simulink model "A3_Multi_DC_bus"  (R2022b)
settings: Solver=ode4  StartTime=0.0  StopTime=tdist2  FixedStep=ts  RelTol=1e-3
undefined symbols (not defined in the file): C, C_bc_ESS, C_bc_PV, C_bc_SC, C_SC_set, Cf, f0, fc, fc1, fv, Gf, Idcbase, Idcbase1, Idcbase2, Ilim, J, Ki_c1, Ki_v, Kp_c1, Kp_v, L_bc_ESS, L_bc_PV, L_bc_SC, L_line_ESS, L_line_PV, Lf, Plim_ESS, Plim_PV, Plim_PV1, Plim_PV2, Plim_SC, Pnom, Pset_ESS, Pset_inv, Pset_load, Pset_PV, Pset_PV1, Pset_PV2, Pset_SC, Qset_inv, R1_line_PV, R2_line_PV, R_bc_ESS, R_bc_PV, R_bc_SC, R_line_ESS, R_line_PV, R_line_SC, Rf, Rg, Sbase, sps, Stotal, tdist1, tdist2, tESSconnect, tPVconnect, ts, tSCconnect, V1 ... (+19)
libraries: spsSeriesRLCBranchLib x20, spsVoltageMeasurementLib x12, spsCurrentMeasurementLib x10, cstblocks x10, spsControlledVoltageSourceLib x9, spsPWMGeneratorDCDCLib x5, spsTwoQuadrantDCDCConverterLib x5, simulink_extras x5, spsBreakerLib x4, spsThreePhaseVIMeasurementLib x3, spsabctoAlphaBetaZeroLib x3, spsThreePhaseSeriesRLCBranchLib x3
(part 2 of 2)

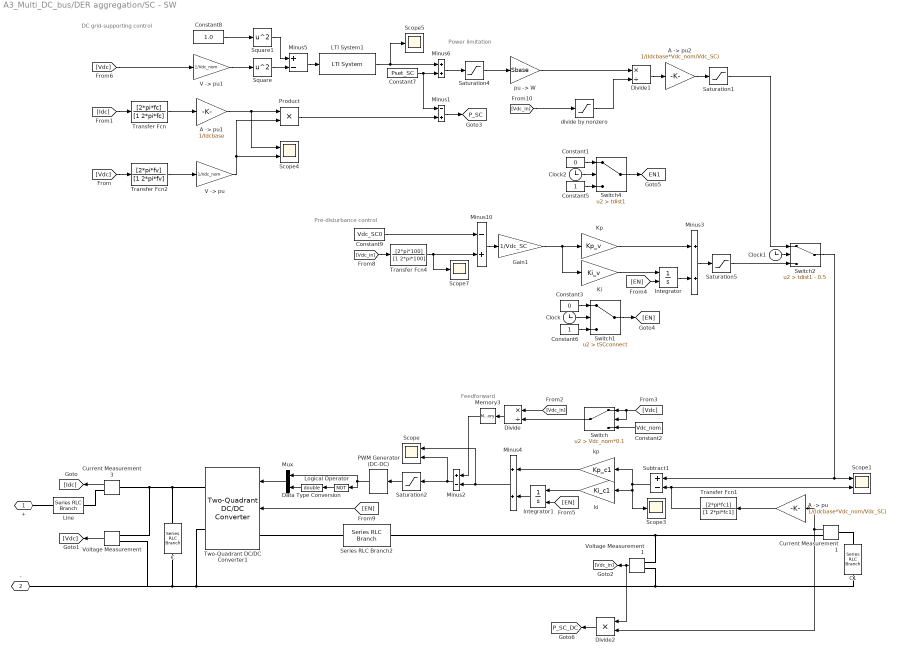
== system A3_Multi_DC_bus/DER aggregation/SC - SW ==
  note: Power limitation
  note: Pre-disturbance control
  note: DC grid-supporting control
  note: Feedforward
  "A -> pu" : Gain  Gain=1/(Idcbase*Vdc_nom/Vdc_SC)
  "A -> pu1" : Gain  Gain=1/Idcbase
  "A -> pu2" : Gain  Gain=1/(Idcbase*Vdc_nom/Vdc_SC)
  C : spsSeriesRLCBranchLib/Series RLC Branch  LConnTagsString=__new0  RConnTagsString=__new0  BranchType=C  Resistance=0.001  Inductance=L_line_PV  SetiL0=off  InitialCurrent=0  Capacitance=C_bc_SC  Setx0=on  InitialVoltage=Vdc_nom  Measurements=None
  C1 : spsSeriesRLCBranchLib/Series RLC Branch  LConnTagsString=__new0  RConnTagsString=__new0  BranchType=C  Resistance=0.001  Inductance=L_line_PV  SetiL0=off  InitialCurrent=0  Capacitance=C_SC_set  Setx0=on  InitialVoltage=Vdc_SC0  Measurements=None
  Clock : Clock
  Clock1 : Clock
  Clock2 : Clock
  Constant1 : Constant  Value=0
  Constant2 : Constant  Value=Vdc_nom
  Constant3 : Constant  Value=0
  Constant5 : Constant
  Constant6 : Constant
  Constant7 : Constant  Value=Pset_SC
  Constant8 : Constant  Value=1.0
  Constant9 : Constant  Value=Vdc_SC0
  Current Measurement1 : spsCurrentMeasurementLib/Current Measurement  PhasorSimulation=off  OutputType=Complex  PSBequivalent=0
  Current Measurement3 : spsCurrentMeasurementLib/Current Measurement  PhasorSimulation=off  OutputType=Complex  PSBequivalent=0
  Data Type Conversion : DataTypeConversion  OutDataTypeStr=double  SaturateOnIntegerOverflow=off  RndMeth=Floor
  Divide : Product  Inputs=*/
  Divide1 : Product  Inputs=*/
  Divide2 : Product  Inputs=**
  Gain1 : Gain  Gain=1/Vdc_SC
  Integrator : Integrator  ExternalReset=level hold  UpperSaturationLimit=1.5  LowerSaturationLimit=-0.5
  Integrator1 : Integrator  ExternalReset=level hold  LimitOutput=on  UpperSaturationLimit=1  LowerSaturationLimit=-1
  Ki : Gain  Gain=Ki_v
  Kp : Gain  Gain=Kp_v
  LTI System1 : cstblocks/LTI System  sys=T_SC1  IC=[]
  Line : spsSeriesRLCBranchLib/Series RLC Branch  LConnTagsString=__new0  RConnTagsString=__new0  BranchType=R  Resistance=R_line_SC  Inductance=L_line_ESS  SetiL0=off  InitialCurrent=0  Capacitance=1e-6  Setx0=off  InitialVoltage=0  Measurements=None
  Logical Operator : Logic  Operator=NOT  AllPortsSameDT=off  OutDataTypeStr=boolean
  Memory3 : Memory
  Minus1 : Sum  Inputs=-+
  Minus10 : Sum  Inputs=-+
  Minus2 : Sum  Inputs=+-
  Minus3 : Sum
  Minus4 : Sum
  Minus5 : Sum  Inputs=+-
  Minus6 : Sum
  Mux : Mux  Inputs=2
  PWM Generator (DC-DC) : spsPWMGeneratorDCDCLib/PWM Generator (DC-DC)  Fsw=fw  Ts=0
  Product : Product
  Saturation1 : Saturate  UpperLimit=1.0  LowerLimit=-1.0
  Saturation2 : Saturate  UpperLimit=1  LowerLimit=0
  Saturation4 : Saturate  UpperLimit=Plim_SC  LowerLimit=-Plim_SC
  Saturation5 : Saturate  UpperLimit=1.0  LowerLimit=-1.0
  Scope : Scope  NumInputPorts=2
  Scope1 : Scope  NumInputPorts=2
  Scope3 : Scope
  Scope4 : Scope  NumInputPorts=2
  Scope5 : Scope
  Scope7 : Scope
  Series RLC Branch2 : spsSeriesRLCBranchLib/Series RLC Branch  LConnTagsString=__new0  RConnTagsString=__new0  BranchType=RL  Resistance=R_bc_SC  Inductance=L_bc_SC  SetiL0=off  InitialCurrent=Pset_SC*Idcbase*Vdc_nom/Vdc_PV  Capacitance=1e-6  Setx0=off  InitialVoltage=0  Measurements=None
  Square : Math  Operator=square
  Square1 : Math  Operator=square
  Subtract1 : Sum  Inputs=+-
  Switch : Switch  Criteria=u2 > Threshold  Threshold=Vdc_nom*0.1  SaturateOnIntegerOverflow=off  InputSameDT=off
  Switch1 : Switch  Criteria=u2 > Threshold  Threshold=tSCconnect  SaturateOnIntegerOverflow=off  InputSameDT=off
  Switch2 : Switch  Criteria=u2 > Threshold  Threshold=tdist1 - 0.5  SaturateOnIntegerOverflow=off  InputSameDT=off
  Switch4 : Switch  Criteria=u2 > Threshold  Threshold=tdist1  SaturateOnIntegerOverflow=off  InputSameDT=off
  Transfer Fcn : TransferFcn  Numerator=[2*pi*fc]  Denominator=[1 2*pi*fc]
  Transfer Fcn1 : TransferFcn  Numerator=[2*pi*fc1]  Denominator=[1 2*pi*fc1]
  Transfer Fcn2 : TransferFcn  Numerator=[2*pi*fv]  Denominator=[1 2*pi*fv]
  Transfer Fcn4 : TransferFcn  Numerator=[2*pi*100]  Denominator=[1 2*pi*100]
  Two-Quadrant DC/DC Converter1 : spsTwoQuadrantDCDCConverterLib/Two-Quadrant DC//DC Converter  ModelType=Switching devices  Ron=1e-4  Rs=1e6  Cs=inf  Vforward=[0,0]  Ron_Diode=1e-3  Rs_Diode=1e6  Cs_Diode=inf  Vf_Diode=1e-3  Rs_CurrentSource=inf  Ron_ACsource=1e-3
      settings: LibrarySourceBlock=|
      | sps_lib/Power Electronics/Two-Quadrant
      | DC//DC Converter
  "V -> pu" : Gain  Gain=1/Vdc_nom
  "V -> pu1" : Gain  Gain=1/Vdc_nom
  Voltage Measurement : spsVoltageMeasurementLib/Voltage Measurement  PhasorSimulation=off  OutputType=Complex  PSBequivalent=0
  Voltage Measurement1 : spsVoltageMeasurementLib/Voltage Measurement  PhasorSimulation=off  OutputType=Complex  PSBequivalent=0
  divide by nonzero : Saturate  UpperLimit=1e6  LowerLimit=1e-6
  ki : Gain  Gain=Ki_c1
  kp : Gain  Gain=Kp_c1
  "pu -> W" : Gain  Gain=Sbase
  + : PMIOPort  Side=Left
  - : PMIOPort  Port=2  Side=Right
  tag scope: EN1=global, P_SC=global, P_SC_DC=global
  wires:
  Constant1/1 -> Switch4/1
  Switch4/1 -> [EN1]
  Clock2/1 -> Switch4/2
  Constant5/1 -> Switch4/3
  Saturation5/1 -> Switch2/3
  Minus1/1 -> [P_SC]
  Saturation4/1 -> "pu -> W"/1
  Subtract1/1 -> ki/1, Scope3/1, kp/1
  Minus6/1 -> Saturation4/1
  Divide1/1 -> "A -> pu2"/1
  divide by nonzero/1 -> Divide1/2
  "pu -> W"/1 -> Divide1/1
  "A -> pu2"/1 -> Saturation1/1
  Clock1/1 -> Switch2/2
  Minus10/1 -> Gain1/1
  [Vdc_in] -> Transfer Fcn4/1
  Constant9/1 -> Minus10/1
  Transfer Fcn4/1 -> Minus10/2, Scope7/1
  [Idc] -> Transfer Fcn/1
  Voltage Measurement/1 -> [Vdc]
  Current Measurement3/1 -> [Idc]
  [EN] -> Two-Quadrant DC/DC Converter1/2
  Current Measurement1/1 -> Divide2/2, "A -> pu"/1
  Transfer Fcn1/1 -> Subtract1/2, Scope1/2
  Product/1 -> Minus1/2
  Switch/1 -> Divide/2
  Constant2/1 -> Switch/3
  [Vdc_in] -> Divide/1
  Divide/1 -> Memory3/1
  Voltage Measurement1/1 -> Divide2/1, [Vdc_in]
  [Vdc] -> Switch/2, Switch/1
  Minus3/1 -> Saturation5/1
  Saturation1/1 -> Switch2/1
  Ki/1 -> Integrator/1
  Integrator/1 -> Minus3/2
  Kp/1 -> Minus3/1
  kp/1 -> Minus4/1
  Integrator1/1 -> Minus4/2
  ki/1 -> Integrator1/1
  Clock/1 -> Switch1/2
  Switch1/1 -> [EN]
  Constant3/1 -> Switch1/1
  Constant6/1 -> Switch1/3
  [EN] -> Integrator/2
  [EN] -> Integrator1/2
  Constant8/1 -> Square1/1
  Square/1 -> Minus5/2
  Square1/1 -> Minus5/1
  Minus5/1 -> LTI System1/1
  Constant7/1 -> Minus6/2, Minus1/1
  LTI System1/1 -> Minus6/1, Scope5/1
  [Vdc] -> "V -> pu1"/1
  "V -> pu1"/1 -> Square/1
  "V -> pu"/1 -> Product/2, Scope4/2
  "A -> pu1"/1 -> Scope4/1, Product/1
  [Vdc] -> Transfer Fcn2/1
  Minus4/1 -> Minus2/2, Scope/1
  Gain1/1 -> Kp/1, Ki/1
  Minus2/1 -> Scope/2, Saturation2/1
  Transfer Fcn/1 -> "A -> pu1"/1
  Transfer Fcn2/1 -> "V -> pu"/1
  "A -> pu"/1 -> Transfer Fcn1/1
  Memory3/1 -> Minus2/1
  Data Type Conversion/1 -> Mux/2
  Saturation2/1 -> PWM Generator (DC-DC)/1
  PWM Generator (DC-DC)/1 -> Mux/1, Logical Operator/1
  Logical Operator/1 -> Data Type Conversion/1
  Mux/1 -> Two-Quadrant DC/DC Converter1/1
  [Vdc_in] -> divide by nonzero/1
  Divide2/1 -> [P_SC_DC]
  Switch2/1 -> Subtract1/1, Scope1/1
  connections:
  C/RConn1 -- -/RConn1 -- Voltage Measurement/LConn2 -- Two-Quadrant DC/DC Converter1/RConn2 -- C1/RConn1 -- Voltage Measurement1/LConn2
  Two-Quadrant DC/DC Converter1/LConn1 -- Series RLC Branch2/LConn1
  C1/LConn1 -- Current Measurement1/LConn1
  Series RLC Branch2/RConn1 -- Voltage Measurement1/LConn1 -- Current Measurement1/RConn1
  Current Measurement3/RConn1 -- Line/RConn1
  Current Measurement3/LConn1 -- Voltage Measurement/LConn1 -- Two-Quadrant DC/DC Converter1/RConn1 -- C/LConn1
  Line/LConn1 -- +/RConn1

== system A3_Multi_DC_bus/Desired (using causalized Ti)/Int ==
  In : Inport
  Constant6 : Constant  Value=2*pi
  Initial : InitialCondition  Value=0
  Integrator1 : Integrator  ExternalReset=rising  InitialConditionSource=external  InitialCondition=sps.Phase_Init*pi/180  ShowStatePort=on
  Relational Operator : RelationalOperator  Operator=>  OutDataTypeStr=boolean  InputSameDT=off
  Subtract : Sum  Inputs=+-
  wt : Outport
  wires:
  Integrator1/1 -> wt/1
  Initial/1 -> Integrator1/3
  In/1 -> Integrator1/1
  Relational Operator/1 -> Integrator1/2
  Subtract/1 -> Initial/1
  Integrator1/State -> Relational Operator/1, Subtract/1
  Constant6/1 -> Relational Operator/2, Subtract/2

== system A3_Multi_DC_bus/Desired (using causalized Ti)/Inv Tr ==
  wt : Inport
  dq : Inport  Port=2
  Fcn : Fcn  Expr=u[1]*cos(u[3]) - u[2]*sin(u[3])
  Fcn1 : Fcn  Expr=u[1]*sin(u[3]) + u[2]*cos(u[3])
  Mux : Mux  Inputs=2
  Mux2 : Mux  Inputs=[2 1]
  Mux3 : Mux  Inputs=[2 1]
  albe : Outport
  wires:
  Fcn1/1 -> Mux/2
  wt/1 -> Mux2/2, Mux3/2
  Fcn/1 -> Mux/1
  Mux/1 -> albe/1
  dq/1 -> Mux2/1, Mux3/1
  Mux2/1 -> Fcn/1
  Mux3/1 -> Fcn1/1

== system A3_Multi_DC_bus/Subsystem/Int ==
  In : Inport
  Constant6 : Constant  Value=2*pi
  Initial : InitialCondition  Value=0
  Integrator1 : Integrator  ExternalReset=rising  InitialConditionSource=external  InitialCondition=sps.Phase_Init*pi/180  ShowStatePort=on
  Relational Operator : RelationalOperator  Operator=>  OutDataTypeStr=boolean  InputSameDT=off
  Subtract : Sum  Inputs=+-
  Out : Outport
  wires:
  Integrator1/1 -> Out/1
  Initial/1 -> Integrator1/3
  In/1 -> Integrator1/1
  Relational Operator/1 -> Integrator1/2
  Subtract/1 -> Initial/1
  Integrator1/State -> Relational Operator/1, Subtract/1
  Constant6/1 -> Relational Operator/2, Subtract/2

== system A3_Multi_DC_bus/Subsystem2/Int ==
  In : Inport
  Constant6 : Constant  Value=2*pi
  Initial : InitialCondition  Value=0
  Integrator1 : Integrator  ExternalReset=rising  InitialConditionSource=external  InitialCondition=sps.Phase_Init*pi/180  ShowStatePort=on
  Relational Operator : RelationalOperator  Operator=>  OutDataTypeStr=boolean  InputSameDT=off
  Subtract : Sum  Inputs=+-
  Out : Outport
  wires:
  Integrator1/1 -> Out/1
  Initial/1 -> Integrator1/3
  In/1 -> Integrator1/1
  Relational Operator/1 -> Integrator1/2
  Subtract/1 -> Initial/1
  Integrator1/State -> Relational Operator/1, Subtract/1
  Constant6/1 -> Relational Operator/2, Subtract/2

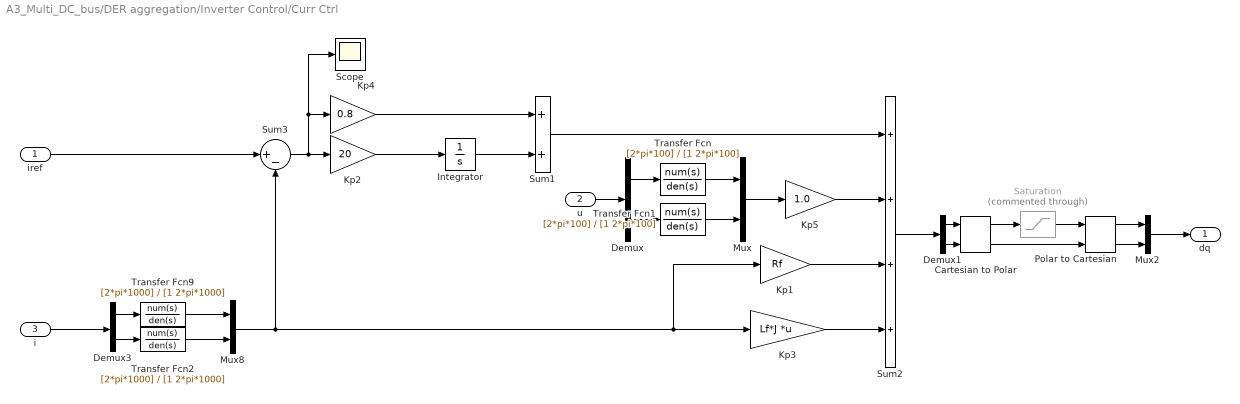
== system A3_Multi_DC_bus/DER aggregation/Inverter Control/Curr Ctrl ==
  iref : Inport
  "u " : Inport  Port=2
  i : Inport  Port=3
  Cartesian to Polar : simulink_extras/Transformations/Cartesian to Polar
  Demux : Demux  Outputs=2
  Demux1 : Demux  Outputs=2
  Demux3 : Demux  Outputs=2
  Integrator : Integrator  InitialCondition=[1 0]
  Kp1 : Gain  Gain=Rf  SaturateOnIntegerOverflow=on  OutDataTypeStr=Inherit: Same as input  ParamDataTypeStr=Inherit: Same as input
  Kp2 : Gain  Gain=20  SaturateOnIntegerOverflow=on  OutDataTypeStr=Inherit: Same as input  ParamDataTypeStr=Inherit: Same as input
  Kp3 : Gain  Gain=Lf*J  Multiplication=Matrix(K*u)  SaturateOnIntegerOverflow=on  OutDataTypeStr=Inherit: Same as input  ParamDataTypeStr=Inherit: Same as input
  Kp4 : Gain  Gain=0.8  SaturateOnIntegerOverflow=on  OutDataTypeStr=Inherit: Same as input  ParamDataTypeStr=Inherit: Same as input
  Kp5 : Gain  Gain=1.0  SaturateOnIntegerOverflow=on  OutDataTypeStr=Inherit: Same as input  ParamDataTypeStr=Inherit: Same as input
  Mux : Mux  Inputs=2
  Mux2 : Mux  Inputs=2
  Mux8 : Mux  Inputs=2
  Polar to Cartesian : simulink_extras/Transformations/Polar to Cartesian
  Saturation : Saturate  Commented=through  UpperLimit=1.5  LowerLimit=0
  Scope : Scope
  Sum1 : Sum
  Sum2 : Sum  Inputs=++++
  Sum3 : Sum  Inputs=|+-
  Transfer Fcn : TransferFcn  Numerator=[2*pi*100]  Denominator=[1 2*pi*100]
  Transfer Fcn1 : TransferFcn  Numerator=[2*pi*100]  Denominator=[1 2*pi*100]
  Transfer Fcn2 : TransferFcn  Numerator=[2*pi*1000]  Denominator=[1 2*pi*1000]
  Transfer Fcn9 : TransferFcn  Numerator=[2*pi*1000]  Denominator=[1 2*pi*1000]
  dq : Outport
  wires:
  Demux3/2 -> Transfer Fcn2/1
  i/1 -> Demux3/1
  Demux3/1 -> Transfer Fcn9/1
  Transfer Fcn9/1 -> Mux8/1
  Transfer Fcn2/1 -> Mux8/2
  iref/1 -> Sum3/1
  Saturation/1 -> Polar to Cartesian/1
  Polar to Cartesian/1 -> Mux2/1
  Sum2/1 -> Demux1/1
  Demux1/1 -> Cartesian to Polar/1
  Cartesian to Polar/1 -> Saturation/1
  Cartesian to Polar/2 -> Polar to Cartesian/2
  Polar to Cartesian/2 -> Mux2/2
  Demux1/2 -> Cartesian to Polar/2
  Transfer Fcn/1 -> Mux/1
  Transfer Fcn1/1 -> Mux/2
  Demux/2 -> Transfer Fcn1/1
  Demux/1 -> Transfer Fcn/1
  Mux/1 -> Kp5/1
  Kp5/1 -> Sum2/2
  "u "/1 -> Demux/1
  Kp3/1 -> Sum2/4
  Kp1/1 -> Sum2/3
  Mux2/1 -> dq/1
  Kp2/1 -> Integrator/1
  Mux8/1 -> Kp3/1, Kp1/1, Sum3/2
  Integrator/1 -> Sum1/2
  Kp4/1 -> Sum1/1
  Sum3/1 -> Kp2/1, Kp4/1, Scope/1
  Sum1/1 -> Sum2/1

== system A3_Multi_DC_bus/DER aggregation/Inverter Control/Curr T ==
  abc : Inport
  In2 : Inport  Port=2
  Demux : Demux  Outputs=3
  Mux1 : Mux  Inputs=2
  Subsystem : Subsystem
  Terminator2 : Terminator
  abc to Alpha-Beta-Zero : spsabctoAlphaBetaZeroLib/abc to Alpha-Beta-Zero
  dq : Outport
  wires:
  In2/1 -> Subsystem/2(wt)
  Mux1/1 -> Subsystem/1(albe)
  abc/1 -> abc to Alpha-Beta-Zero/1
  Demux/2 -> Mux1/2
  Demux/1 -> Mux1/1
  Demux/3 -> Terminator2/1
  abc to Alpha-Beta-Zero/1 -> Demux/1
  Subsystem/1(dq) -> dq/1

== system A3_Multi_DC_bus/DER aggregation/Inverter Control/Curr in T ==
  abc : Inport
  In2 : Inport  Port=2
  Demux : Demux  Outputs=3
  Mux1 : Mux  Inputs=2
  Subsystem : Subsystem
  Terminator2 : Terminator
  abc to Alpha-Beta-Zero : spsabctoAlphaBetaZeroLib/abc to Alpha-Beta-Zero
  dq : Outport
  wires:
  Subsystem/1(dq) -> dq/1
  In2/1 -> Subsystem/2(wt)
  Mux1/1 -> Subsystem/1(albe)
  abc/1 -> abc to Alpha-Beta-Zero/1
  Demux/2 -> Mux1/2
  Demux/1 -> Mux1/1
  Demux/3 -> Terminator2/1
  abc to Alpha-Beta-Zero/1 -> Demux/1

== system A3_Multi_DC_bus/DER aggregation/Inverter Control/Int ==
  In : Inport
  Constant6 : Constant  Value=2*pi
  Initial : InitialCondition  Value=0
  Integrator1 : Integrator  ExternalReset=rising  InitialConditionSource=external  InitialCondition=sps.Phase_Init*pi/180  ShowStatePort=on
  Relational Operator : RelationalOperator  Operator=>  OutDataTypeStr=boolean  InputSameDT=off
  Subtract : Sum  Inputs=+-
  Out : Outport
  wires:
  Integrator1/1 -> Out/1
  Initial/1 -> Integrator1/3
  In/1 -> Integrator1/1
  Relational Operator/1 -> Integrator1/2
  Subtract/1 -> Initial/1
  Integrator1/State -> Relational Operator/1, Subtract/1
  Constant6/1 -> Relational Operator/2, Subtract/2

== system A3_Multi_DC_bus/DER aggregation/Inverter Control/Inv Tr ==
  dq : Inport
  wt : Inport  Port=2
  Fcn : Fcn  Expr=u[1]*cos(u[3]) - u[2]*sin(u[3])
  Fcn1 : Fcn  Expr=u[1]*sin(u[3]) + u[2]*cos(u[3])
  Mux : Mux  Inputs=2
  Mux2 : Mux  Inputs=[2 1]
  Mux3 : Mux  Inputs=[2 1]
  albe : Outport
  wires:
  Fcn1/1 -> Mux/2
  wt/1 -> Mux2/2, Mux3/2
  Fcn/1 -> Mux/1
  Mux/1 -> albe/1
  dq/1 -> Mux2/1, Mux3/1
  Mux2/1 -> Fcn/1
  Mux3/1 -> Fcn1/1

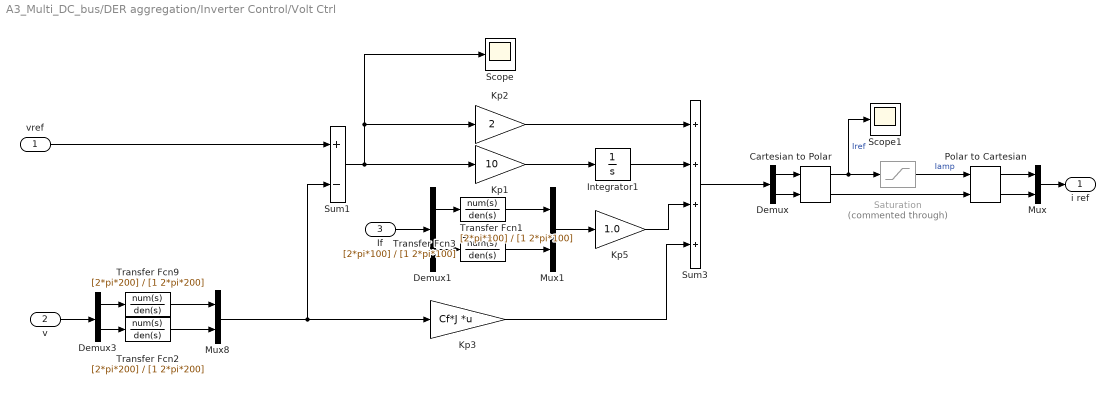
== system A3_Multi_DC_bus/DER aggregation/Inverter Control/Volt Ctrl ==
  vref : Inport
  v : Inport  Port=2
  If : Inport  Port=3
  Cartesian to Polar : simulink_extras/Transformations/Cartesian to Polar
  Demux : Demux  Outputs=2
  Demux1 : Demux  Outputs=2
  Demux3 : Demux  Outputs=2
  Integrator1 : Integrator  InitialCondition=[0 0]
  Kp1 : Gain  Gain=10  SaturateOnIntegerOverflow=on  OutDataTypeStr=Inherit: Same as input  ParamDataTypeStr=Inherit: Same as input
  Kp2 : Gain  Gain=2  SaturateOnIntegerOverflow=on  OutDataTypeStr=Inherit: Same as input  ParamDataTypeStr=Inherit: Same as input
  Kp3 : Gain  Gain=Cf*J  Multiplication=Matrix(K*u)  SaturateOnIntegerOverflow=on  OutDataTypeStr=Inherit: Same as input  ParamDataTypeStr=Inherit: Same as input
  Kp5 : Gain  Gain=1.0  SaturateOnIntegerOverflow=on  OutDataTypeStr=Inherit: Same as input  ParamDataTypeStr=Inherit: Same as input
  Mux : Mux  Inputs=2
  Mux1 : Mux  Inputs=2
  Mux8 : Mux  Inputs=2
  Polar to Cartesian : simulink_extras/Transformations/Polar to Cartesian
  Saturation : Saturate  Commented=through  UpperLimit=Ilim  LowerLimit=0
  Scope : Scope
  Scope1 : Scope
  Sum1 : Sum  Inputs=+-
  Sum3 : Sum  Inputs=++++
  Transfer Fcn1 : TransferFcn  Numerator=[2*pi*100]  Denominator=[1 2*pi*100]
  Transfer Fcn2 : TransferFcn  Numerator=[2*pi*200]  Denominator=[1 2*pi*200]
  Transfer Fcn3 : TransferFcn  Numerator=[2*pi*100]  Denominator=[1 2*pi*100]
  Transfer Fcn9 : TransferFcn  Numerator=[2*pi*200]  Denominator=[1 2*pi*200]
  i ref : Outport
  wires:
  vref/1 -> Sum1/1
  Demux1/2 -> Transfer Fcn3/1
  Demux/1 -> Cartesian to Polar/1
  Mux8/1 -> Sum1/2, Kp3/1
  Cartesian to Polar/2 -> Polar to Cartesian/2
  Demux/2 -> Cartesian to Polar/2
  Saturation/1 -> Polar to Cartesian/1  "Iamp"
  Integrator1/1 -> Sum3/2
  Mux1/1 -> Kp5/1
  Kp1/1 -> Integrator1/1
  Transfer Fcn1/1 -> Mux1/1
  Kp2/1 -> Sum3/1
  Transfer Fcn3/1 -> Mux1/2
  If/1 -> Demux1/1
  Demux1/1 -> Transfer Fcn1/1
  Kp5/1 -> Sum3/3
  Sum3/1 -> Demux/1
  Sum1/1 -> Kp2/1, Scope/1, Kp1/1
  Polar to Cartesian/1 -> Mux/1
  Polar to Cartesian/2 -> Mux/2
  Mux/1 -> i ref/1
  Cartesian to Polar/1 -> Saturation/1, Scope1/1  "Iref"
  Transfer Fcn2/1 -> Mux8/2
  Transfer Fcn9/1 -> Mux8/1
  Demux3/2 -> Transfer Fcn2/1
  Demux3/1 -> Transfer Fcn9/1
  v/1 -> Demux3/1
  Kp3/1 -> Sum3/4

== system A3_Multi_DC_bus/DER aggregation/Inverter Control/Volt T ==
  abc : Inport
  In2 : Inport  Port=2
  Demux : Demux  Outputs=3
  Mux1 : Mux  Inputs=2
  Subsystem : Subsystem
  Terminator2 : Terminator
  abc to Alpha-Beta-Zero : spsabctoAlphaBetaZeroLib/abc to Alpha-Beta-Zero
  dq : Outport
  wires:
  Subsystem/1(dq) -> dq/1
  abc to Alpha-Beta-Zero/1 -> Demux/1
  Demux/3 -> Terminator2/1
  Demux/1 -> Mux1/1
  Demux/2 -> Mux1/2
  abc/1 -> abc to Alpha-Beta-Zero/1
  Mux1/1 -> Subsystem/1(albe)
  In2/1 -> Subsystem/2(wt)

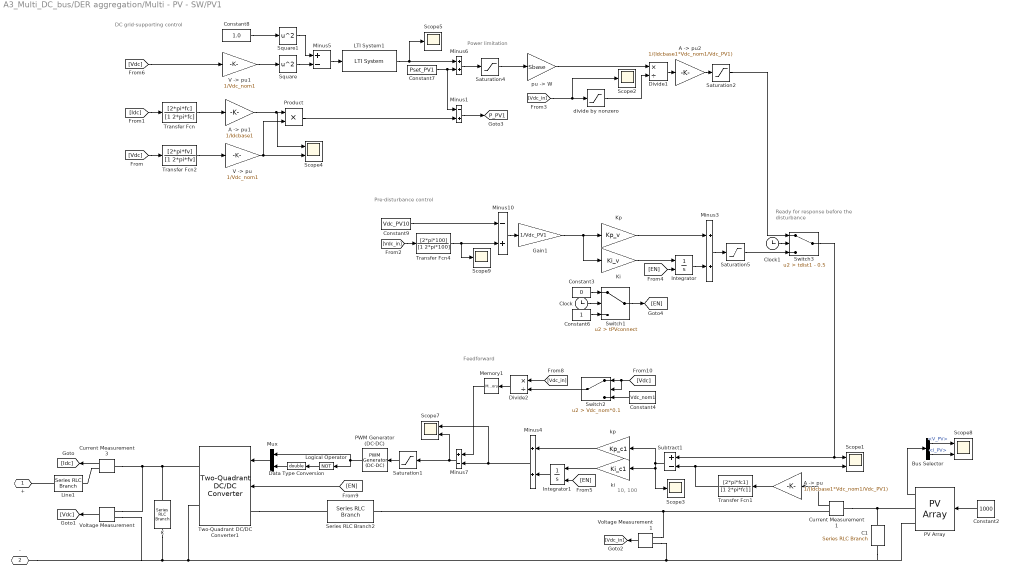
== system A3_Multi_DC_bus/DER aggregation/Multi - PV - SW/PV1 ==
  note: Ready for response
      | before the disturbance
  note: Feedforward
  note: DC grid-supporting control
  note: 10, 100
  note: Pre-disturbance control
  note: Power limitation
  "A -> pu" : Gain  Gain=1/(Idcbase1*Vdc_nom1/Vdc_PV1)
  "A -> pu1" : Gain  Gain=1/Idcbase1
  "A -> pu2" : Gain  Gain=1/(Idcbase1*Vdc_nom1/Vdc_PV1)
  Bus Selector : BusSelector  OutputSignals=V_PV,I_PV
  C : spsSeriesRLCBranchLib/Series RLC Branch  LConnTagsString=__new0  RConnTagsString=__new0  BranchType=C  Resistance=0.001  Inductance=L_line_PV  SetiL0=off  InitialCurrent=0  Capacitance=C_bc_PV  Setx0=on  InitialVoltage=Vdc_nom1  Measurements=None
  C1 : spsSeriesRLCBranchLib/Series RLC Branch  LConnTagsString=__new0  RConnTagsString=__new0  BranchType=C  Resistance=0.001  Inductance=L_line_PV  SetiL0=off  InitialCurrent=0  Capacitance=C_bc_PV  Setx0=on  InitialVoltage=Vdc_PV10  Measurements=None
  Clock : Clock
  Clock1 : Clock
  Constant2 : Constant  Value=1000
  Constant3 : Constant  Value=0
  Constant4 : Constant  Value=Vdc_nom1
  Constant6 : Constant
  Constant7 : Constant  Value=Pset_PV1
  Constant8 : Constant  Value=1.0
  Constant9 : Constant  Value=Vdc_PV10
  Current Measurement1 : spsCurrentMeasurementLib/Current Measurement  PhasorSimulation=off  OutputType=Complex  PSBequivalent=0
  Current Measurement3 : spsCurrentMeasurementLib/Current Measurement  PhasorSimulation=off  OutputType=Complex  PSBequivalent=0
  Data Type Conversion : DataTypeConversion  OutDataTypeStr=double  SaturateOnIntegerOverflow=off  RndMeth=Floor
  Divide1 : Product  Inputs=*/
  Divide2 : Product  Inputs=*/
  Gain1 : Gain  Gain=1/Vdc_PV1
  Integrator : Integrator  ExternalReset=level hold  UpperSaturationLimit=1.5  LowerSaturationLimit=-0.5
  Integrator1 : Integrator  ExternalReset=level hold  LimitOutput=on  UpperSaturationLimit=1  LowerSaturationLimit=-1
  Ki : Gain  Gain=Ki_v
  Kp : Gain  Gain=Kp_v
  LTI System1 : cstblocks/LTI System  sys=T_PV1  IC=[]
  Line1 : spsSeriesRLCBranchLib/Series RLC Branch  LConnTagsString=__new0  RConnTagsString=__new0  BranchType=R  Resistance=R1_line_PV  Inductance=L_line_PV  SetiL0=off  InitialCurrent=0  Capacitance=1e-6  Setx0=off  InitialVoltage=0  Measurements=None
  Logical Operator : Logic  Operator=NOT  AllPortsSameDT=off  OutDataTypeStr=boolean
  Memory1 : Memory
  Minus1 : Sum  Inputs=-+
  Minus10 : Sum  Inputs=-+
  Minus3 : Sum
  Minus4 : Sum
  Minus5 : Sum  Inputs=+-
  Minus6 : Sum
  Minus7 : Sum  Inputs=+-
  Mux : Mux  Inputs=2
  PV Array : spsPVArrayLib/PV Array  Npar=408  Nser=4  PlotType=array @ 1000 W/m2 & specified temperatures  S_vec="[ 1000  500  100 ]"  Temp_C_vec=40  ModuleName=SunPower SPR-315E-WHT-D  PlotWhenSelected=off  Pm=315.072  Ncell=96  Voc=64.6  Isc=6.14  Vm=54.7  Im=5.76  beta_Voc_pc=-0.2727  alpha_Isc_pc=0.061743  beta_Voc=-0.17616  alpha_Isc=0.003791  IL=6.1461  I0=6.5067e-12  nI=0.95071  Rsh=430.0666  Rs=0.43041  RobustModel=on  RobustCellTemperature=40  BAL=off  Tc=1e-6  Tfilter=5e-5
  PWM Generator (DC-DC) : spsPWMGeneratorDCDCLib/PWM Generator (DC-DC)  Fsw=fw  Ts=0
  Product : Product
  Saturation1 : Saturate  UpperLimit=1  LowerLimit=0
  Saturation2 : Saturate  UpperLimit=1.0  LowerLimit=-1.0
  Saturation4 : Saturate  UpperLimit=Plim_PV1  LowerLimit=0
  Saturation5 : Saturate  UpperLimit=1.0  LowerLimit=-1.0
  Scope{1,4,7..8} (4 alike) : Scope  NumInputPorts=2
  Scope{2..3,5,9} (4 alike) : Scope
  Series RLC Branch2 : spsSeriesRLCBranchLib/Series RLC Branch  LConnTagsString=__new0  RConnTagsString=__new0  BranchType=RL  Resistance=R_bc_PV  Inductance=L_bc_PV  SetiL0=off  InitialCurrent=Pset_PV*Idcbase*Vdc_nom/Vdc_PV  Capacitance=1e-6  Setx0=off  InitialVoltage=0  Measurements=None
  Square : Math  Operator=square
  Square1 : Math  Operator=square
  Subtract1 : Sum  Inputs=+-
  Switch1 : Switch  Criteria=u2 > Threshold  Threshold=tPVconnect  SaturateOnIntegerOverflow=off  InputSameDT=off
  Switch2 : Switch  Criteria=u2 > Threshold  Threshold=Vdc_nom*0.1  SaturateOnIntegerOverflow=off  InputSameDT=off
  Switch3 : Switch  Criteria=u2 > Threshold  Threshold=tdist1 - 0.5  SaturateOnIntegerOverflow=off  InputSameDT=off
  Transfer Fcn : TransferFcn  Numerator=[2*pi*fc]  Denominator=[1 2*pi*fc]
  Transfer Fcn1 : TransferFcn  Numerator=[2*pi*fc1]  Denominator=[1 2*pi*fc1]
  Transfer Fcn2 : TransferFcn  Numerator=[2*pi*fv]  Denominator=[1 2*pi*fv]
  Transfer Fcn4 : TransferFcn  Numerator=[2*pi*100]  Denominator=[1 2*pi*100]
  Two-Quadrant DC/DC Converter1 : spsTwoQuadrantDCDCConverterLib/Two-Quadrant DC//DC Converter  ModelType=Switching devices  Ron=1e-4  Rs=1e6  Cs=inf  Vforward=[0,0]  Ron_Diode=1e-3  Rs_Diode=1e6  Cs_Diode=inf  Vf_Diode=1e-3  Rs_CurrentSource=inf  Ron_ACsource=1e-3
      settings: LibrarySourceBlock=|
      | sps_lib/Power Electronics/Two-Quadrant
      | DC//DC Converter
  "V -> pu" : Gain  Gain=1/Vdc_nom1
  "V -> pu1" : Gain  Gain=1/Vdc_nom1
  Voltage Measurement : spsVoltageMeasurementLib/Voltage Measurement  PhasorSimulation=off  OutputType=Complex  PSBequivalent=0
  Voltage Measurement1 : spsVoltageMeasurementLib/Voltage Measurement  PhasorSimulation=off  OutputType=Complex  PSBequivalent=0
  divide by nonzero : Saturate  UpperLimit=1e6  LowerLimit=1e-6
  ki : Gain  Gain=Ki_c1
  kp : Gain  Gain=Kp_c1
  "pu -> W" : Gain  Gain=Sbase
  + : PMIOPort  Side=Left
  - : PMIOPort  Port=2  Side=Right
  tag scope: P_PV1=global
  wires:
  Minus4/1 -> Minus7/2, Scope7/1
  Clock/1 -> Switch1/2
  Constant3/1 -> Switch1/1
  Constant6/1 -> Switch1/3
  Switch1/1 -> [EN]
  Saturation2/1 -> Switch3/1
  Saturation5/1 -> Switch3/3
  Clock1/1 -> Switch3/2
  Minus1/1 -> [P_PV1]
  Saturation4/1 -> "pu -> W"/1
  Minus6/1 -> Saturation4/1
  Divide1/1 -> "A -> pu2"/1
  divide by nonzero/1 -> Divide1/2
  "pu -> W"/1 -> Divide1/1
  "A -> pu2"/1 -> Saturation2/1
  Transfer Fcn4/1 -> Minus10/2, Scope9/1
  [Vdc_in] -> Transfer Fcn4/1
  Minus10/1 -> Gain1/1
  Constant9/1 -> Minus10/1
  Constant2/1 -> PV Array/1
  Bus Selector/2 -> Scope8/2  "<I_PV>"
  Bus Selector/1 -> Scope8/1  "<V_PV>"
  PV Array/1 -> Bus Selector/1
  Minus7/1 -> Saturation1/1, Scope7/2
  Memory1/1 -> Minus7/1
  Divide2/1 -> Memory1/1
  Switch3/1 -> Subtract1/1, Scope1/1
  [Vdc_in] -> Divide2/1
  [Vdc] -> Switch2/1, Switch2/2
  Constant4/1 -> Switch2/3
  Switch2/1 -> Divide2/2
  [Idc] -> Transfer Fcn/1
  Voltage Measurement/1 -> [Vdc]
  Current Measurement3/1 -> [Idc]
  [EN] -> Two-Quadrant DC/DC Converter1/2
  Minus3/1 -> Saturation5/1
  Ki/1 -> Integrator/1
  Integrator/1 -> Minus3/2
  Kp/1 -> Minus3/1
  kp/1 -> Minus4/1
  Integrator1/1 -> Minus4/2
  ki/1 -> Integrator1/1
  Subtract1/1 -> kp/1, ki/1, Scope3/1
  [EN] -> Integrator/2
  [EN] -> Integrator1/2
  Constant8/1 -> Square1/1
  Square/1 -> Minus5/2
  Square1/1 -> Minus5/1
  Minus5/1 -> LTI System1/1
  Constant7/1 -> Minus6/2, Minus1/1
  LTI System1/1 -> Minus6/1, Scope5/1
  [Vdc] -> "V -> pu1"/1
  "V -> pu1"/1 -> Square/1
  "V -> pu"/1 -> Product/2, Scope4/2
  "A -> pu1"/1 -> Scope4/1, Product/1
  [Vdc] -> Transfer Fcn2/1
  Gain1/1 -> Kp/1, Ki/1
  Transfer Fcn/1 -> "A -> pu1"/1
  Transfer Fcn2/1 -> "V -> pu"/1
  Transfer Fcn1/1 -> Scope1/2, Subtract1/2
  "A -> pu"/1 -> Transfer Fcn1/1
  Logical Operator/1 -> Data Type Conversion/1
  Saturation1/1 -> PWM Generator (DC-DC)/1
  PWM Generator (DC-DC)/1 -> Mux/1, Logical Operator/1
  Data Type Conversion/1 -> Mux/2
  Product/1 -> Minus1/2
  Mux/1 -> Two-Quadrant DC/DC Converter1/1
  [Vdc_in] -> divide by nonzero/1, Scope2/1
  Voltage Measurement1/1 -> [Vdc_in]
  Current Measurement1/1 -> "A -> pu"/1
  connections:
  C1/RConn1 -- PV Array/RConn2 -- Voltage Measurement1/LConn2 -- Two-Quadrant DC/DC Converter1/RConn2 -- -/RConn1 -- Voltage Measurement/LConn2 -- C/RConn1
  Two-Quadrant DC/DC Converter1/LConn1 -- Series RLC Branch2/LConn1
  Voltage Measurement1/LConn1 -- Series RLC Branch2/RConn1 -- Current Measurement1/RConn1
  Two-Quadrant DC/DC Converter1/RConn1 -- C/LConn1 -- Current Measurement3/LConn1 -- Voltage Measurement/LConn1
  Current Measurement3/RConn1 -- Line1/RConn1
  Current Measurement1/LConn1 -- C1/LConn1 -- PV Array/RConn1
  Line1/LConn1 -- +/RConn1

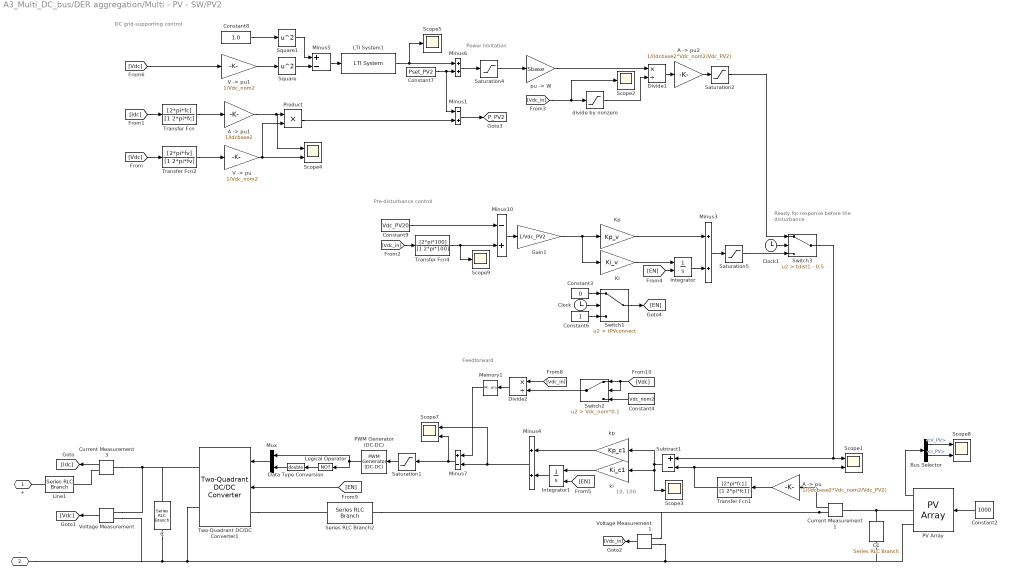
== system A3_Multi_DC_bus/DER aggregation/Multi - PV - SW/PV2 ==
  note: Power limitation
  note: Pre-disturbance control
  note: 10, 100
  note: DC grid-supporting control
  note: Feedforward
  note: Ready for response
      | before the disturbance
  "A -> pu" : Gain  Gain=1/(Idcbase2*Vdc_nom2/Vdc_PV2)
  "A -> pu1" : Gain  Gain=1/Idcbase2
  "A -> pu2" : Gain  Gain=1/(Idcbase2*Vdc_nom2/Vdc_PV2)
  Bus Selector : BusSelector  OutputSignals=V_PV,I_PV
  C : spsSeriesRLCBranchLib/Series RLC Branch  LConnTagsString=__new0  RConnTagsString=__new0  BranchType=C  Resistance=0.001  Inductance=L_line_PV  SetiL0=off  InitialCurrent=0  Capacitance=C_bc_PV  Setx0=on  InitialVoltage=Vdc_nom2  Measurements=None
  C1 : spsSeriesRLCBranchLib/Series RLC Branch  LConnTagsString=__new0  RConnTagsString=__new0  BranchType=C  Resistance=0.001  Inductance=L_line_PV  SetiL0=off  InitialCurrent=0  Capacitance=C_bc_PV  Setx0=on  InitialVoltage=Vdc_PV20  Measurements=None
  Clock : Clock
  Clock1 : Clock
  Constant2 : Constant  Value=1000
  Constant3 : Constant  Value=0
  Constant4 : Constant  Value=Vdc_nom2
  Constant6 : Constant
  Constant7 : Constant  Value=Pset_PV2
  Constant8 : Constant  Value=1.0
  Constant9 : Constant  Value=Vdc_PV20
  Current Measurement1 : spsCurrentMeasurementLib/Current Measurement  PhasorSimulation=off  OutputType=Complex  PSBequivalent=0
  Current Measurement3 : spsCurrentMeasurementLib/Current Measurement  PhasorSimulation=off  OutputType=Complex  PSBequivalent=0
  Data Type Conversion : DataTypeConversion  OutDataTypeStr=double  SaturateOnIntegerOverflow=off  RndMeth=Floor
  Divide1 : Product  Inputs=*/
  Divide2 : Product  Inputs=*/
  Gain1 : Gain  Gain=1/Vdc_PV2
  Integrator : Integrator  ExternalReset=level hold  UpperSaturationLimit=1.5  LowerSaturationLimit=-0.5
  Integrator1 : Integrator  ExternalReset=level hold  LimitOutput=on  UpperSaturationLimit=1  LowerSaturationLimit=-1
  Ki : Gain  Gain=Ki_v
  Kp : Gain  Gain=Kp_v
  LTI System1 : cstblocks/LTI System  sys=T_PV2  IC=[]
  Line1 : spsSeriesRLCBranchLib/Series RLC Branch  LConnTagsString=__new0  RConnTagsString=__new0  BranchType=R  Resistance=R2_line_PV  Inductance=L_line_PV  SetiL0=off  InitialCurrent=0  Capacitance=1e-6  Setx0=off  InitialVoltage=0  Measurements=None
  Logical Operator : Logic  Operator=NOT  AllPortsSameDT=off  OutDataTypeStr=boolean
  Memory1 : Memory
  Minus1 : Sum  Inputs=-+
  Minus10 : Sum  Inputs=-+
  Minus3 : Sum
  Minus4 : Sum
  Minus5 : Sum  Inputs=+-
  Minus6 : Sum
  Minus7 : Sum  Inputs=+-
  Mux : Mux  Inputs=2
  PV Array : spsPVArrayLib/PV Array  Npar=175  Nser=4  PlotType=array @ 1000 W/m2 & specified temperatures  S_vec="[ 1000  500  100 ]"  Temp_C_vec=40  ModuleName=SunPower SPR-315E-WHT-D  PlotWhenSelected=off  Pm=315.072  Ncell=96  Voc=64.6  Isc=6.14  Vm=54.7  Im=5.76  beta_Voc_pc=-0.2727  alpha_Isc_pc=0.061743  beta_Voc=-0.17616  alpha_Isc=0.003791  IL=6.1461  I0=6.5067e-12  nI=0.95071  Rsh=430.0666  Rs=0.43041  RobustModel=on  RobustCellTemperature=40  BAL=off  Tc=1e-6  Tfilter=5e-5
  PWM Generator (DC-DC) : spsPWMGeneratorDCDCLib/PWM Generator (DC-DC)  Fsw=fw  Ts=0
  Product : Product
  Saturation1 : Saturate  UpperLimit=1  LowerLimit=0
  Saturation2 : Saturate  UpperLimit=1.0  LowerLimit=-1.0
  Saturation4 : Saturate  UpperLimit=Plim_PV2  LowerLimit=0
  Saturation5 : Saturate  UpperLimit=1.0  LowerLimit=-1.0
  Scope{1,4,7..8} (4 alike) : Scope  NumInputPorts=2
  Scope{2..3,5,9} (4 alike) : Scope
  Series RLC Branch2 : spsSeriesRLCBranchLib/Series RLC Branch  LConnTagsString=__new0  RConnTagsString=__new0  BranchType=RL  Resistance=R_bc_PV  Inductance=L_bc_PV  SetiL0=off  InitialCurrent=Pset_PV*Idcbase*Vdc_nom/Vdc_PV  Capacitance=1e-6  Setx0=off  InitialVoltage=0  Measurements=None
  Square : Math  Operator=square
  Square1 : Math  Operator=square
  Subtract1 : Sum  Inputs=+-
  Switch1 : Switch  Criteria=u2 > Threshold  Threshold=tPVconnect  SaturateOnIntegerOverflow=off  InputSameDT=off
  Switch2 : Switch  Criteria=u2 > Threshold  Threshold=Vdc_nom*0.1  SaturateOnIntegerOverflow=off  InputSameDT=off
  Switch3 : Switch  Criteria=u2 > Threshold  Threshold=tdist1 - 0.5  SaturateOnIntegerOverflow=off  InputSameDT=off
  Transfer Fcn : TransferFcn  Numerator=[2*pi*fc]  Denominator=[1 2*pi*fc]
  Transfer Fcn1 : TransferFcn  Numerator=[2*pi*fc1]  Denominator=[1 2*pi*fc1]
  Transfer Fcn2 : TransferFcn  Numerator=[2*pi*fv]  Denominator=[1 2*pi*fv]
  Transfer Fcn4 : TransferFcn  Numerator=[2*pi*100]  Denominator=[1 2*pi*100]
  Two-Quadrant DC/DC Converter1 : spsTwoQuadrantDCDCConverterLib/Two-Quadrant DC//DC Converter  ModelType=Switching devices  Ron=1e-4  Rs=1e6  Cs=inf  Vforward=[0,0]  Ron_Diode=1e-3  Rs_Diode=1e6  Cs_Diode=inf  Vf_Diode=1e-3  Rs_CurrentSource=inf  Ron_ACsource=1e-3
      settings: LibrarySourceBlock=|
      | sps_lib/Power Electronics/Two-Quadrant
      | DC//DC Converter
  "V -> pu" : Gain  Gain=1/Vdc_nom2
  "V -> pu1" : Gain  Gain=1/Vdc_nom2
  Voltage Measurement : spsVoltageMeasurementLib/Voltage Measurement  PhasorSimulation=off  OutputType=Complex  PSBequivalent=0
  Voltage Measurement1 : spsVoltageMeasurementLib/Voltage Measurement  PhasorSimulation=off  OutputType=Complex  PSBequivalent=0
  divide by nonzero : Saturate  UpperLimit=1e6  LowerLimit=1e-6
  ki : Gain  Gain=Ki_c1
  kp : Gain  Gain=Kp_c1
  "pu -> W" : Gain  Gain=Sbase
  + : PMIOPort  Side=Left
  - : PMIOPort  Port=2  Side=Right
  tag scope: P_PV2=global
  wires:
  Current Measurement1/1 -> "A -> pu"/1
  Voltage Measurement1/1 -> [Vdc_in]
  [Vdc_in] -> Scope2/1, divide by nonzero/1
  Mux/1 -> Two-Quadrant DC/DC Converter1/1
  Product/1 -> Minus1/2
  Data Type Conversion/1 -> Mux/2
  PWM Generator (DC-DC)/1 -> Logical Operator/1, Mux/1
  Saturation1/1 -> PWM Generator (DC-DC)/1
  Logical Operator/1 -> Data Type Conversion/1
  "A -> pu"/1 -> Transfer Fcn1/1
  Transfer Fcn1/1 -> Subtract1/2, Scope1/2
  Transfer Fcn2/1 -> "V -> pu"/1
  Transfer Fcn/1 -> "A -> pu1"/1
  Gain1/1 -> Ki/1, Kp/1
  [Vdc] -> Transfer Fcn2/1
  "A -> pu1"/1 -> Product/1, Scope4/1
  "V -> pu"/1 -> Scope4/2, Product/2
  "V -> pu1"/1 -> Square/1
  [Vdc] -> "V -> pu1"/1
  LTI System1/1 -> Scope5/1, Minus6/1
  Constant7/1 -> Minus1/1, Minus6/2
  Minus5/1 -> LTI System1/1
  Square1/1 -> Minus5/1
  Square/1 -> Minus5/2
  Constant8/1 -> Square1/1
  [EN] -> Integrator1/2
  [EN] -> Integrator/2
  Subtract1/1 -> Scope3/1, ki/1, kp/1
  ki/1 -> Integrator1/1
  Integrator1/1 -> Minus4/2
  kp/1 -> Minus4/1
  Kp/1 -> Minus3/1
  Integrator/1 -> Minus3/2
  Ki/1 -> Integrator/1
  Minus3/1 -> Saturation5/1
  [EN] -> Two-Quadrant DC/DC Converter1/2
  Current Measurement3/1 -> [Idc]
  Voltage Measurement/1 -> [Vdc]
  [Idc] -> Transfer Fcn/1
  Switch2/1 -> Divide2/2
  Constant4/1 -> Switch2/3
  [Vdc] -> Switch2/2, Switch2/1
  [Vdc_in] -> Divide2/1
  Switch3/1 -> Scope1/1, Subtract1/1
  Divide2/1 -> Memory1/1
  Memory1/1 -> Minus7/1
  Minus7/1 -> Scope7/2, Saturation1/1
  PV Array/1 -> Bus Selector/1
  Bus Selector/1 -> Scope8/1  "<V_PV>"
  Bus Selector/2 -> Scope8/2  "<I_PV>"
  Constant2/1 -> PV Array/1
  Constant9/1 -> Minus10/1
  Minus10/1 -> Gain1/1
  [Vdc_in] -> Transfer Fcn4/1
  Transfer Fcn4/1 -> Scope9/1, Minus10/2
  "A -> pu2"/1 -> Saturation2/1
  "pu -> W"/1 -> Divide1/1
  divide by nonzero/1 -> Divide1/2
  Divide1/1 -> "A -> pu2"/1
  Minus6/1 -> Saturation4/1
  Saturation4/1 -> "pu -> W"/1
  Minus1/1 -> [P_PV2]
  Clock1/1 -> Switch3/2
  Saturation5/1 -> Switch3/3
  Saturation2/1 -> Switch3/1
  Switch1/1 -> [EN]
  Constant6/1 -> Switch1/3
  Constant3/1 -> Switch1/1
  Clock/1 -> Switch1/2
  Minus4/1 -> Scope7/1, Minus7/2
  connections:
  Current Measurement1/LConn1 -- C1/LConn1 -- PV Array/RConn1
  Current Measurement3/RConn1 -- Line1/RConn1
  Voltage Measurement/LConn1 -- Current Measurement3/LConn1 -- C/LConn1 -- Two-Quadrant DC/DC Converter1/RConn1
  Current Measurement1/RConn1 -- Series RLC Branch2/RConn1 -- Voltage Measurement1/LConn1
  Two-Quadrant DC/DC Converter1/LConn1 -- Series RLC Branch2/LConn1
  C1/RConn1 -- PV Array/RConn2 -- Voltage Measurement1/LConn2 -- Two-Quadrant DC/DC Converter1/RConn2 -- C/RConn1 -- Voltage Measurement/LConn2 -- -/RConn1
  Line1/LConn1 -- +/RConn1

== system A3_Multi_DC_bus/DER aggregation/Inverter Control/Curr T/Subsystem ==
  note: d = al*cos(wt) + be*sin(wt)
  note: q = -al*sin(wt) + be*cos(wt)
  albe : Inport
  wt : Inport  Port=2
  Fcn : Fcn  Expr=u[1]*cos(u[3]) + u[2]*sin(u[3])
  Fcn1 : Fcn  Expr=-u[1]*sin(u[3]) + u[2]*cos(u[3])
  Mux : Mux  Inputs=2
  Mux2 : Mux  Inputs=[2 1]
  Mux3 : Mux  Inputs=[2 1]
  dq : Outport
  wires:
  Fcn1/1 -> Mux/2
  wt/1 -> Mux2/2, Mux3/2
  Fcn/1 -> Mux/1
  Mux/1 -> dq/1
  albe/1 -> Mux2/1, Mux3/1
  Mux2/1 -> Fcn/1
  Mux3/1 -> Fcn1/1

== system A3_Multi_DC_bus/DER aggregation/Inverter Control/Curr in T/Subsystem ==
  note: d = al*cos(wt) + be*sin(wt)
  note: q = -al*sin(wt) + be*cos(wt)
  albe : Inport
  wt : Inport  Port=2
  Fcn : Fcn  Expr=u[1]*cos(u[3]) + u[2]*sin(u[3])
  Fcn1 : Fcn  Expr=-u[1]*sin(u[3]) + u[2]*cos(u[3])
  Mux : Mux  Inputs=2
  Mux2 : Mux  Inputs=[2 1]
  Mux3 : Mux  Inputs=[2 1]
  dq : Outport
  wires:
  Fcn1/1 -> Mux/2
  wt/1 -> Mux2/2, Mux3/2
  Fcn/1 -> Mux/1
  Mux/1 -> dq/1
  albe/1 -> Mux2/1, Mux3/1
  Mux2/1 -> Fcn/1
  Mux3/1 -> Fcn1/1

== system A3_Multi_DC_bus/DER aggregation/Inverter Control/Volt T/Subsystem ==
  note: q = -al*sin(wt) + be*cos(wt)
  note: d = al*cos(wt) + be*sin(wt)
  albe : Inport
  wt : Inport  Port=2
  Fcn : Fcn  Expr=u[1]*cos(u[3]) + u[2]*sin(u[3])
  Fcn1 : Fcn  Expr=-u[1]*sin(u[3]) + u[2]*cos(u[3])
  Mux : Mux  Inputs=2
  Mux2 : Mux  Inputs=[2 1]
  Mux3 : Mux  Inputs=[2 1]
  dq : Outport
  wires:
  Mux3/1 -> Fcn1/1
  Mux2/1 -> Fcn/1
  albe/1 -> Mux3/1, Mux2/1
  Mux/1 -> dq/1
  Fcn/1 -> Mux/1
  wt/1 -> Mux3/2, Mux2/2
  Fcn1/1 -> Mux/2
